simulink model "FOC_Model_IM"  (R2016a)
settings: Solver=ode45  StartTime=0.0  StopTime=10.0  RelTol=1e-3
undefined symbols (not defined in the file): ctrl_sat, DiscIntNeverNeededParam
libraries: powerlib x4, simulink x2
settings Model: Creator=Copy864  LastModifiedBy=Copy864

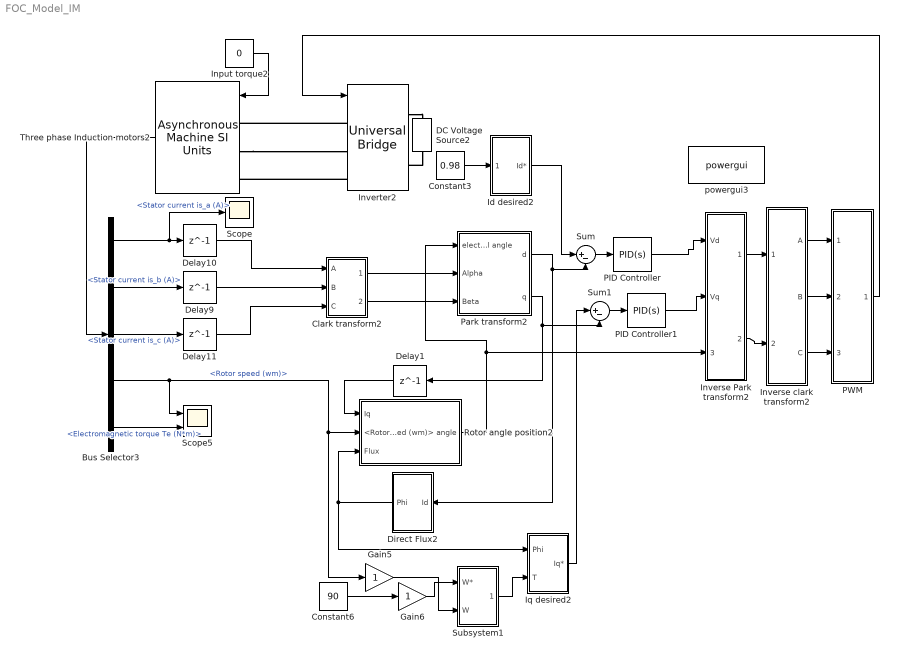
== system FOC_Model_IM ==
  Bus Selector3 : BusSelector  OutputSignals=Stator measurements.Stator current is_a (A),Stator measurements.Stator current is_b (A),Stator measurements.Stator current is_c (A),Mechanical.Rotor speed (wm),Mechanical.Electromagnetic torque Te (N*m)
  Clark transform2 : Subsystem
  Constant3 : Constant  Value=0.98
  Constant6 : Constant  Value=90
  DC Voltage Source2 : powerlib/Electrical Sources/DC Voltage Source  Amplitude=500  Measurements=None
  Delay1 : Delay  DelayLength=1  InitialCondition=0  SampleTime=0.0001
  Delay10 : Delay  DelayLength=1  InitialCondition=0
  Delay11 : Delay  DelayLength=1  InitialCondition=0
  Delay9 : Delay  DelayLength=1  InitialCondition=0
  Direct Flux2 : Subsystem
  Gain5 : Gain
  Gain6 : Gain
  Id desired2 : Subsystem
  Input torque2 : Constant  Value=0
  Inverse Park transform2 : Subsystem
  Inverse clark transform2 : Subsystem
  Inverter2 : powerlib/Power Electronics/Universal Bridge  Arms=3  SnubberResistance=1e5  SnubberCapacitance=inf  Device=IGBT / Diodes  Ron=1e-3  Lon=0  ForwardVoltages="[  0  0  ]"  ForwardVoltage=0  GTOparameters=[ 10e-6 , 20e-6 ]  IGBTparameters=[ 1e-6 , 2e-6 ]  Measurements=Device voltages  Measurements_2=None  converterType=Rectifier
  Iq desired2 : Subsystem
  PID Controller : simulink/Continuous/PID Controller  Controller=PID  TimeDomain=Continuous-time  SampleTime=-1  IntegratorMethod=Forward Euler  FilterMethod=Forward Euler  Form=Parallel  UseFilter=on  ControllerParametersSource=internal  P=5000  I=200  D=0  N=100  InitialConditionSource=internal  InitialConditionForIntegrator=0  InitialConditionForFilter=0  ExternalReset=none  LimitOutput=off  UpperSaturationLimit=inf  LowerSaturationLimit=-inf  LinearizeAsGain=on  AntiWindupMode=none  Kb=1  TrackingMode=off  Kt=1  PParamMin=[]  PParamMax=[]  IParamMin=[]  IParamMax=[]  DParamMin=[]  DParamMax=[]  NParamMin=[]  NParamMax=[]  KbParamMin=[]  KbParamMax=[]  KtParamMin=[]  KtParamMax=[]  POutMin=[]  POutMax=[]  IOutMin=[]  IOutMax=[]  DOutMin=[]  DOutMax=[]  NOutMin=[]  NOutMax=[]  KbOutMin=[]  KbOutMax=[]  KtOutMin=[]  KtOutMax=[]  IntegratorOutMin=[]  IntegratorOutMax=[]  FilterOutMin=[]  FilterOutMax=[]  SumOutMin=[]  SumOutMax=[]  SumI1OutMin=[]  SumI1OutMax=[]  SumI2OutMin=[]  SumI2OutMax=[]  SumI3OutMin=[]  SumI3OutMax=[]  SumDOutMin=[]  SumDOutMax=[]  SaturationOutMin=[]  SaturationOutMax=[]  IntegratorContinuousStateAttributes=''  IntegratorStateMustResolveToSignalObject=off  IntegratorRTWStateStorageClass=Auto  FilterContinuousStateAttributes=''  FilterStateMustResolveToSignalObject=off  FilterRTWStateStorageClass=Auto  DifferentiatorICPrevScaledInput=0  DifferentiatorOutMin=[]  DifferentiatorOutMax=[]
  PID Controller1 : simulink/Continuous/PID Controller  Controller=PID  TimeDomain=Continuous-time  SampleTime=-1  IntegratorMethod=Forward Euler  FilterMethod=Forward Euler  Form=Parallel  UseFilter=on  ControllerParametersSource=internal  P=5000  I=200  D=0  N=100  InitialConditionSource=internal  InitialConditionForIntegrator=0  InitialConditionForFilter=0  ExternalReset=none  LimitOutput=off  UpperSaturationLimit=inf  LowerSaturationLimit=-inf  LinearizeAsGain=on  AntiWindupMode=none  Kb=1  TrackingMode=off  Kt=1  PParamMin=[]  PParamMax=[]  IParamMin=[]  IParamMax=[]  DParamMin=[]  DParamMax=[]  NParamMin=[]  NParamMax=[]  KbParamMin=[]  KbParamMax=[]  KtParamMin=[]  KtParamMax=[]  POutMin=[]  POutMax=[]  IOutMin=[]  IOutMax=[]  DOutMin=[]  DOutMax=[]  NOutMin=[]  NOutMax=[]  KbOutMin=[]  KbOutMax=[]  KtOutMin=[]  KtOutMax=[]  IntegratorOutMin=[]  IntegratorOutMax=[]  FilterOutMin=[]  FilterOutMax=[]  SumOutMin=[]  SumOutMax=[]  SumI1OutMin=[]  SumI1OutMax=[]  SumI2OutMin=[]  SumI2OutMax=[]  SumI3OutMin=[]  SumI3OutMax=[]  SumDOutMin=[]  SumDOutMax=[]  SaturationOutMin=[]  SaturationOutMax=[]  IntegratorContinuousStateAttributes=''  IntegratorStateMustResolveToSignalObject=off  IntegratorRTWStateStorageClass=Auto  FilterContinuousStateAttributes=''  FilterStateMustResolveToSignalObject=off  FilterRTWStateStorageClass=Auto  DifferentiatorICPrevScaledInput=0  DifferentiatorOutMin=[]  DifferentiatorOutMax=[]
  PWM : Subsystem
  Park transform2 : Subsystem
  Rotor angle position2 : Subsystem
  Scope : Scope
  Scope5 : Scope  NumInputPorts=2
  Subsystem1 : Subsystem
  Sum : Sum  Inputs=|+-
  Sum1 : Sum  Inputs=|+-
  Three phase Induction motors2 : powerlib/Machines/Asynchronous Machine SI Units  RotorType=Squirrel-cage  PresetModel=No  MechanicalLoad=Torque Tm  ShowDetailedParameters=on  ReferenceFrame=Rotor  Units=SI  MeasurementBus=off  NominalParameters=[7460 460 60]  Stator=[0.6837 0.004152]  Rotor=[0.451 0.004152]  Cage1=[0.4155 0.002066]  Cage2=[0.4168 0.0003495]  Lm=0.1486  Mechanical=[0.05 0.02791 1]  PolePairs=2  InitialConditions=[1 0 0 0 0 0 0 0]  SimulateSaturation=off  Saturation=[14.03593122, 27.81365428, 53.79336849, 72.68890987, 97.98006896, 148.6815601, 215.7428561, 302.9841135, 428.7778367 ; 230, 322, 414, 460, 506, 552, 598, 644, 690]  LoadFlowParameters=1492000  TsPowergui=0  TsBlock=2*10^-6  IterativeModel=Trapezoidal non iterative  IterativeDiscreteModel=Trapezoidal iterative (alg. loop)  Pmec=1.492e+006
  powergui3 : powerlib/powergui  Priority=1  SimulationMode=Discrete  SolverType=Tustin/Backward Euler (TBE)  SampleTime=2*10^(-6)  frequency=60  SPID=off  DisableSnubberDevices=off  DisableRonSwitches=off  DisableVfSwitches=off  SwTol=0  DisplayEquations=off  Interpol=off  ExternalGateDelay=off  methode=off  Ts=100  FunctionMessages=on  echomessages=off  HookPort=off  EnableUseOfTLC=on  x0status=blocks  frequencyindice=0  Pbase=100e6  ErrMax=1e-4  Iterations=50  UnitsV=kV  UnitsW=MW  buscounter=0  RestoreLinks=warning  ResistiveCurrentMeasurement=off  Frange=[0:2:500]  Ylog=off  Xlog=on  ShowGrid=off  save=off  variable=ZData  structure=0  ZoomFFT=off  StartTime=0.0  cycles=1  DisplayStyle=1  fundamental=60  FreqAxis=off  MaxFrequency=1000  frequencyindicesteady=1  RmsSteady=1  display=off
  wires:
  Three phase Induction motors2/1 -> Bus Selector3/1
  Park transform2/2(q) -> Delay1/1, Sum1/2
  Bus Selector3/2 -> Delay9/1  "<Stator current is_b (A)>"
  Bus Selector3/3 -> Delay11/1  "<Stator current is_c (A)>"
  Clark transform2/2(Beta) -> Park transform2/3(Beta)
  Delay11/1 -> Clark transform2/3(C)
  Bus Selector3/1 -> Scope/1, Delay10/1  "<Stator current is_a (A)>"
  Clark transform2/1(Alpha) -> Park transform2/2(Alpha)
  Delay10/1 -> Clark transform2/1(A)
  Delay9/1 -> Clark transform2/2(B)
  Delay1/1 -> Rotor angle position2/1(Iq)
  Rotor angle position2/1(angle) -> Inverse Park transform2/3(theta), Park transform2/1(electrical angle)
  Park transform2/1(d) -> Sum/2, Direct Flux2/1(Id)
  Direct Flux2/1(Phi) -> Iq desired2/1(Phi), Rotor angle position2/3(Flux)
  Bus Selector3/4 -> Rotor angle position2/2(<Rotor speed (wm)>), Gain5/1, Scope5/1  "<Rotor speed (wm)>"
  Constant3/1 -> Id desired2/1(Phi*)
  Gain5/1 -> Subsystem1/2(W)
  Gain6/1 -> Subsystem1/1(W*)
  Constant6/1 -> Gain6/1
  Subsystem1/1(Te*) -> Iq desired2/2(T)
  Bus Selector3/5 -> Scope5/2  "<Electromagnetic torque Te (N*m)>"
  Input torque2/1 -> Three phase Induction motors2/1
  PID Controller/1 -> Inverse Park transform2/1(Vd)
  Inverse clark transform2/2(B) -> PWM/2(Vb*)
  Inverse clark transform2/1(A) -> PWM/1(Va*)
  Inverse Park transform2/1(Alpha) -> Inverse clark transform2/1(Alpha)
  Inverse Park transform2/2(Beta) -> Inverse clark transform2/2(Beta)
  Sum1/1 -> PID Controller1/1
  Sum/1 -> PID Controller/1
  Inverse clark transform2/3(C) -> PWM/3(Vc*)
  PID Controller1/1 -> Inverse Park transform2/2(Vq)
  PWM/1(Gate) -> Inverter2/1
  Id desired2/1(Id*) -> Sum/1
  Iq desired2/1(Iq*) -> Sum1/1
  connections:
  Three phase Induction motors2/LConn2 -- Inverter2/LConn2
  Inverter2/RConn1 -- DC Voltage Source2/RConn1
  DC Voltage Source2/LConn1 -- Inverter2/RConn2
  Inverter2/LConn1 -- Three phase Induction motors2/LConn1
  Inverter2/LConn3 -- Three phase Induction motors2/LConn3

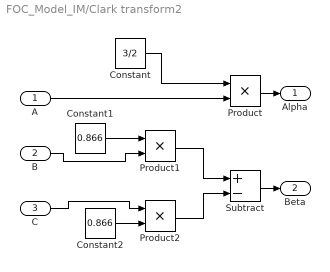
== system FOC_Model_IM/Clark transform2 ==
  A : Inport
  B : Inport  Port=2
  C : Inport  Port=3
  Constant : Constant  Value=3/2
  Constant1 : Constant  Value=0.866
  Constant2 : Constant  Value=0.866
  Product : Product
  Product1 : Product
  Product2 : Product
  Subtract : Sum  Inputs=+-
  Alpha : Outport
  Beta : Outport  Port=2
  wires:
  Product1/1 -> Subtract/1
  Product2/1 -> Subtract/2
  Product/1 -> Alpha/1
  Constant1/1 -> Product1/1
  Constant/1 -> Product/1
  Constant2/1 -> Product2/2
  Subtract/1 -> Beta/1
  C/1 -> Product2/1
  B/1 -> Product1/2
  A/1 -> Product/2

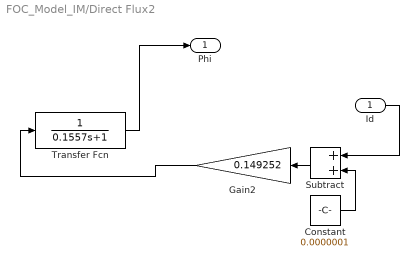
== system FOC_Model_IM/Direct Flux2 ==
  Id : Inport
  Constant : Constant  Value=0.0000001
  Gain2 : Gain  Gain=0.149252
  Subtract : Sum
  Transfer Fcn : TransferFcn  Denominator=[0.1557 1]
  Phi : Outport
  wires:
  Gain2/1 -> Transfer Fcn/1
  Transfer Fcn/1 -> Phi/1
  Id/1 -> Subtract/1
  Subtract/1 -> Gain2/1
  Constant/1 -> Subtract/2

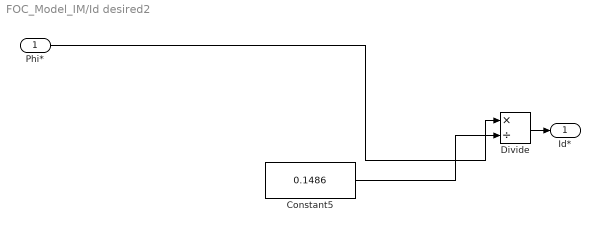
== system FOC_Model_IM/Id desired2 ==
  Phi* : Inport
  Constant5 : Constant  Value=0.1486
  Divide : Product  Inputs=*/
  Id* : Outport
  wires:
  Phi*/1 -> Divide/1
  Divide/1 -> Id*/1
  Constant5/1 -> Divide/2

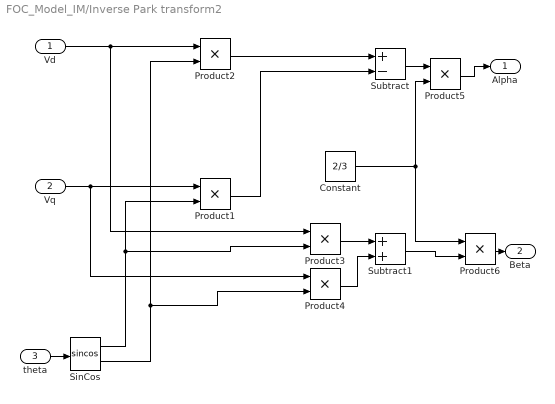
== system FOC_Model_IM/Inverse Park transform2 ==
  Vd : Inport
  Vq : Inport  Port=2
  theta : Inport  Port=3
  Constant : Constant  Value=2/3
  Product{1..6} (6 alike) : Product
  SinCos : Trigonometry  Operator=sincos
  Subtract : Sum  Inputs=+-
  Subtract1 : Sum
  Alpha : Outport
  Beta : Outport  Port=2
  wires:
  SinCos/2 -> Product4/2, Product2/2
  SinCos/1 -> Product3/2, Product1/2
  Vd/1 -> Product3/1, Product2/1
  Vq/1 -> Product4/1, Product1/1
  Product1/1 -> Subtract/2
  Product3/1 -> Subtract1/1
  Product2/1 -> Subtract/1
  theta/1 -> SinCos/1
  Product4/1 -> Subtract1/2
  Subtract/1 -> Product5/1
  Product5/1 -> Alpha/1
  Product6/1 -> Beta/1
  Subtract1/1 -> Product6/2
  Constant/1 -> Product6/1, Product5/2

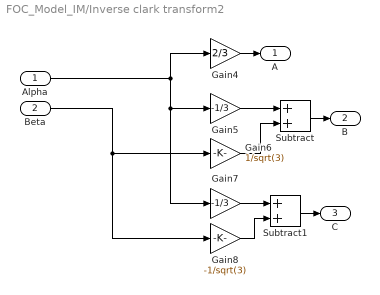
== system FOC_Model_IM/Inverse clark transform2 ==
  Alpha : Inport
  Beta : Inport  Port=2
  Gain4 : Gain  Gain=2/3
  Gain5 : Gain  Gain=-1/3
  Gain6 : Gain  Gain=1/sqrt(3)
  Gain7 : Gain  Gain=-1/3
  Gain8 : Gain  Gain=-1/sqrt(3)
  Subtract : Sum
  Subtract1 : Sum
  A : Outport
  B : Outport  Port=2
  C : Outport  Port=3
  wires:
  Subtract/1 -> B/1
  Alpha/1 -> Gain4/1, Gain7/1, Gain5/1
  Gain5/1 -> Subtract/1
  Subtract1/1 -> C/1
  Gain4/1 -> A/1
  Gain6/1 -> Subtract/2
  Beta/1 -> Gain8/1, Gain6/1
  Gain8/1 -> Subtract1/2
  Gain7/1 -> Subtract1/1

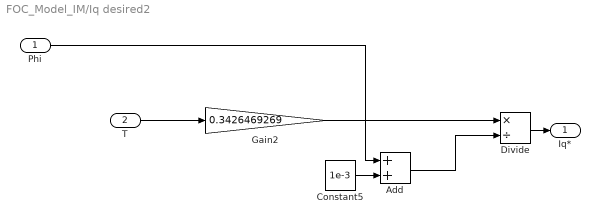
== system FOC_Model_IM/Iq desired2 ==
  Phi : Inport
  T : Inport  Port=2
  Add : Sum
  Constant5 : Constant  Value=1e-3
  Divide : Product  Inputs=*/
  Gain2 : Gain  Gain=0.3426469269
  Iq* : Outport
  wires:
  Add/1 -> Divide/2
  Constant5/1 -> Add/2
  Divide/1 -> Iq*/1
  Gain2/1 -> Divide/1
  Phi/1 -> Add/1
  T/1 -> Gain2/1

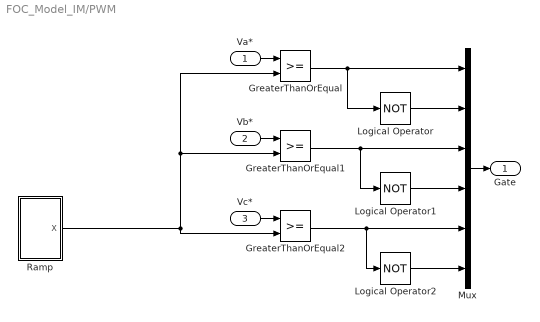
== system FOC_Model_IM/PWM ==
  Va* : Inport
  Vb* : Inport  Port=2
  Vc* : Inport  Port=3
  GreaterThanOrEqual : RelationalOperator  OutDataTypeStr=boolean
  GreaterThanOrEqual1 : RelationalOperator  OutDataTypeStr=boolean
  GreaterThanOrEqual2 : RelationalOperator  OutDataTypeStr=boolean
  Logical Operator : Logic  Operator=NOT  AllPortsSameDT=off  OutDataTypeStr=boolean
  Logical Operator1 : Logic  Operator=NOT  AllPortsSameDT=off  OutDataTypeStr=boolean
  Logical Operator2 : Logic  Operator=NOT  AllPortsSameDT=off  OutDataTypeStr=boolean
  Mux : Mux  Inputs=6
  "Ramp " : Subsystem
  Gate : Outport
  wires:
  Logical Operator/1 -> Mux/2
  Logical Operator1/1 -> Mux/4
  GreaterThanOrEqual1/1 -> Logical Operator1/1, Mux/3
  "Ramp "/1(X) -> GreaterThanOrEqual/2, GreaterThanOrEqual1/2, GreaterThanOrEqual2/2
  Vc*/1 -> GreaterThanOrEqual2/1
  GreaterThanOrEqual2/1 -> Mux/5, Logical Operator2/1
  GreaterThanOrEqual/1 -> Logical Operator/1, Mux/1
  Mux/1 -> Gate/1
  Logical Operator2/1 -> Mux/6
  Va*/1 -> GreaterThanOrEqual/1
  Vb*/1 -> GreaterThanOrEqual1/1

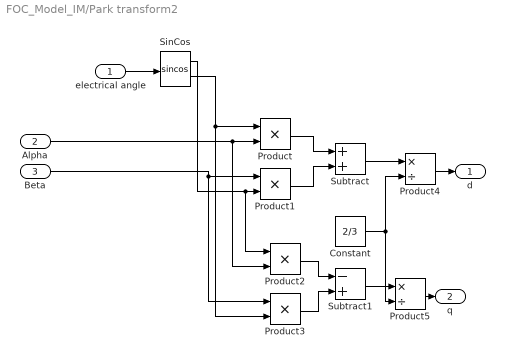
== system FOC_Model_IM/Park transform2 ==
  electrical angle : Inport
  Alpha : Inport  Port=2
  Beta : Inport  Port=3
  Constant : Constant  Value=2/3
  Product{,1..3} (4 alike) : Product
  Product4 : Product  Inputs=*/
  Product5 : Product  Inputs=*/
  SinCos : Trigonometry  Operator=sincos
  Subtract : Sum
  Subtract1 : Sum  Inputs=-+
  d : Outport
  q : Outport  Port=2
  wires:
  electrical angle/1 -> SinCos/1
  SinCos/1 -> Product2/1, Product1/2
  Alpha/1 -> Product2/2, Product/2
  SinCos/2 -> Product/1, Product3/2
  Product3/1 -> Subtract1/2
  Product2/1 -> Subtract1/1
  Beta/1 -> Product3/1, Product1/1
  Product1/1 -> Subtract/2
  Product/1 -> Subtract/1
  Subtract1/1 -> Product5/1
  Subtract/1 -> Product4/1
  Product5/1 -> q/1
  Product4/1 -> d/1
  Constant/1 -> Product5/2, Product4/2

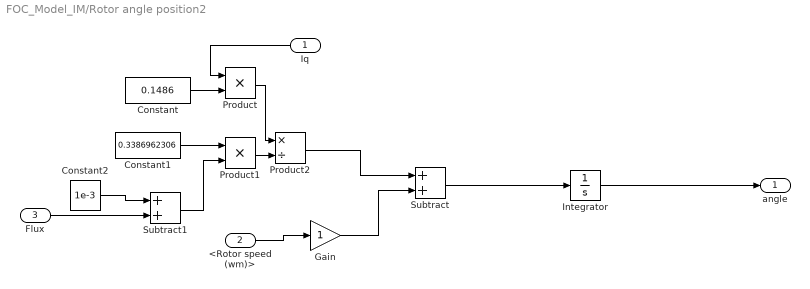
== system FOC_Model_IM/Rotor angle position2 ==
  Iq : Inport
  <Rotor speed (wm)> : Inport  Port=2
  Flux : Inport  Port=3
  Constant : Constant  Value=0.1486
  Constant1 : Constant  Value=0.3386962306
  Constant2 : Constant  Value=1e-3
  Gain : Gain
  Integrator : Integrator  AbsoluteTolerance=2*10^-6  ZeroCross=off
  Product : Product
  Product1 : Product
  Product2 : Product  Inputs=*/
  Subtract : Sum
  Subtract1 : Sum
  angle : Outport
  wires:
  Subtract/1 -> Integrator/1
  Constant/1 -> Product/2
  Constant1/1 -> Product1/1
  Product/1 -> Product2/1
  Gain/1 -> Subtract/2
  Product1/1 -> Product2/2
  Iq/1 -> Product/1
  <Rotor speed (wm)>/1 -> Gain/1
  Integrator/1 -> angle/1
  Product2/1 -> Subtract/1
  Flux/1 -> Subtract1/2
  Subtract1/1 -> Product1/2
  Constant2/1 -> Subtract1/1

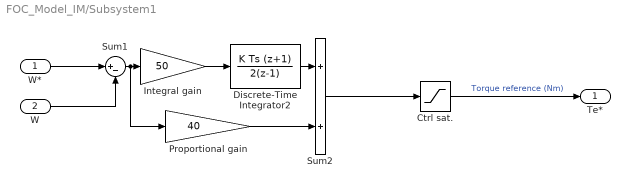
== system FOC_Model_IM/Subsystem1 ==
  W* : Inport
  W : Inport  Port=2
  Ctrl sat. : Saturate  UpperLimit=1e6  LowerLimit=-2000
  Discrete-Time Integrator2 : DiscreteIntegrator  IntegratorMethod=Integration: Trapezoidal  SampleTime=-1  UpperSaturationLimit=ctrl_sat(2)  LowerSaturationLimit=ctrl_sat(1)  ICPrevOutput=DiscIntNeverNeededParam  ICPrevScaledInput=DiscIntNeverNeededParam
  Integral gain : Gain  Gain=50  SaturateOnIntegerOverflow=on  OutDataTypeStr=Inherit: Same as input  ParamDataTypeStr=Inherit: Same as input
  Proportional gain : Gain  Gain=40  SaturateOnIntegerOverflow=on  OutDataTypeStr=Inherit: Same as input  ParamDataTypeStr=Inherit: Same as input
  Sum1 : Sum  Inputs=|+-  SaturateOnIntegerOverflow=on  InputSameDT=on  OutDataTypeStr=Inherit: Same as first input
  Sum2 : Sum  SaturateOnIntegerOverflow=on  InputSameDT=on  OutDataTypeStr=Inherit: Same as first input
  Te* : Outport
  wires:
  Sum2/1 -> Ctrl sat./1
  Integral gain/1 -> Discrete-Time Integrator2/1
  Discrete-Time Integrator2/1 -> Sum2/1
  Sum1/1 -> Integral gain/1, Proportional gain/1
  Proportional gain/1 -> Sum2/2
  W*/1 -> Sum1/1
  W/1 -> Sum1/2
  Ctrl sat./1 -> Te*/1  "Torque reference (Nm)"

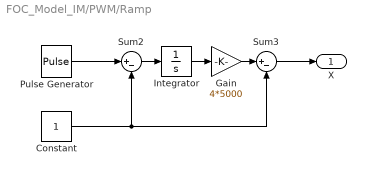
== system FOC_Model_IM/PWM/Ramp  ==
  Constant : Constant
  Gain : Gain  Gain=4*5000
  Integrator : Integrator
  Pulse Generator : DiscretePulseGenerator  PulseType=Time based  Amplitude=2  Period=1/5000  PulseWidth=5
  Sum2 : Sum  Inputs=|+-
  Sum3 : Sum  Inputs=|+-
  X : Outport
  wires:
  Sum3/1 -> X/1
  Gain/1 -> Sum3/1
  Constant/1 -> Sum3/2, Sum2/2
  Integrator/1 -> Gain/1
  Pulse Generator/1 -> Sum2/1
  Sum2/1 -> Integrator/1
